simulink model "ARS1_2connection_k5"  (R2018a)
settings: Solver=VariableStepAuto  StartTime=0.0  StopTime=10.0  RelTol=1e-3
settings Model: Creator=moizh  LastModifiedBy=moizh

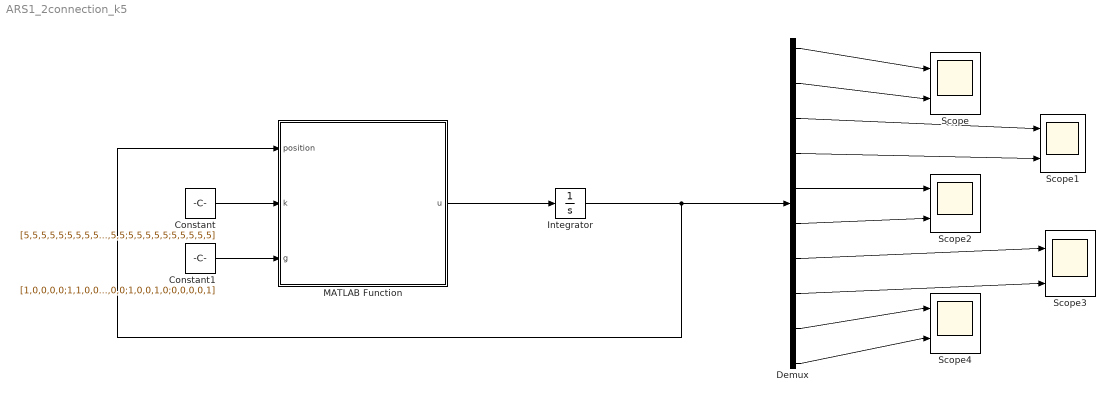
== system ARS1_2connection_k5 ==
  Constant : Constant  Value=[5,5,5,5,5;5,5,5,5,5;5,5,5,5,5;5,5,5,5,5;5,5,5,5,5]
  Constant1 : Constant  Value=[1,0,0,0,0;1,1,0,0,0;0,0,1,0,0;1,0,0,1,0;0,0,0,0,1]
  Demux : Demux  Outputs=10
  Integrator : Integrator  InitialCondition=[0;1.5;0;-1.5;-3;3;-3;0;-3;-3]
  MATLAB Function : MATLAB Function  TreatAsAtomicUnit=on
  Scope{,1..4} (5 alike) : Scope  NumInputPorts=2
  wires:
  Constant/1 -> MATLAB Function/2(k)
  Constant1/1 -> MATLAB Function/3(g)
  MATLAB Function/1(u) -> Integrator/1
  Integrator/1 -> MATLAB Function/1(position), Demux/1
  Demux/1 -> Scope/1
  Demux/2 -> Scope/2
  Demux/3 -> Scope1/1
  Demux/4 -> Scope1/2
  Demux/5 -> Scope2/1
  Demux/6 -> Scope2/2
  Demux/7 -> Scope3/1
  Demux/8 -> Scope3/2
  Demux/9 -> Scope4/1
  Demux/10 -> Scope4/2

== matlab function ARS1_2connection_k5/MATLAB Function ==
  data: position input; u output; k input; g input
function u = fcn(position,k,g)

 
a11 = -g(1,1)*k(1,1)-g(1,2)*k(1,2)-g(1,3)*k(1,3)-g(1,4)*k(1,4)-g(1,5)*k(1,5);
a12 = 0;
a13 = g(1,2)*k(1,2);
a14 = 0;
a15 = g(1,3)*k(1,3);
a16 = 0;
a17 = g(1,4)*k(1,4);
a18 = 0;
a19 = g(1,5)*k(1,5);
a110 = 0;

a21 = 0;
a22 = -g(1,1)*k(1,1)-g(1,2)*k(1,2)-g(1,3)*k(1,3)-g(1,4)*k(1,4)-g(1,5)*k(1,5);
a23 = 0;
a24 = g(1,2)*k(1,2);
a25 = 0;
a26 = g(1,3)*k(1,3);
a27 = 0;
a28 = g(1,4)*k(1,4);
a29 = 0;
a210 = g(1,5)*k(1,5);

a31 = g(2,1)*k(2,1);
a32 = 0;
a33 = -g(2,1)*k(2,1)-g(2,2)*k(2,2)-g(2,3)*k(2,3)-g(2,4)*k(2,4)-g(2,5)*k(2,5);
a34 = 0;
a35 = g(2,3)*k(2,3);
a36 = 0;
a37 = g(2,4)*k(2,4);
a38 = 0;
a39 = g(2,5)*k(2,5);
a310 = 0;

a41 = 0;
a42 = g(2,1)*k(2,1);
a43 = 0;
a44 = -g(2,1)*k(2,1)-g(2,2)*k(2,2)-g(2,3)*k(2,3)-g(2,4)*k(2,4)-g(2,5)*k(2,5);
a45 = 0;
a46 = g(2,3)*k(2,3);
a47 = 0;
a48 = g(2,4)*k(2,4);
a49 = 0;
a410 = g(2,5)*k(2,5);

a51 = g(3,1)*k(3,1);
a52 = 0;
a53 = g(3,2)*k(3,2);
a54 = 0;
a55 = -g(3,1)*k(3,1)-g(3,2)*k(3,2)-g(3,3)*k(3,3)-g(3,4)*k(3,4)-g(3,5)*k(3,5);
a56 = 0;
a57 = g(3,4)*k(3,4);
a58 = 0;
a59 = g(3,5)*k(3,5);
a510 = 0;

a61 = 0;
a62 = g(3,1)*k(3,1);
a63 = 0;
a64 = g(3,2)*k(3,2);
a65 = 0;
a66 = -g(3,1)*k(3,1)-g(3,2)*k(3,2)-g(3,3)*k(3,3)-g(3,4)*k(3,4)-g(3,5)*k(3,5);
a67 = 0;
a68 = g(3,4)*k(3,4);
a69 = 0;
a610 = g(3,5)*k(3,5);

a71 = g(4,1)*k(4,1);
a72 = 0;
a73 = g(4,2)*k(4,2);
a74 = 0;
a75 = g(4,3)*k(4,3);
a76 = 0;
a77 = -g(4,1)*k(4,1)-g(4,2)*k(4,2)-g(4,3)*k(4,3)-g(4,4)*k(4,4)-g(4,5)*k(4,5);
a78 = 0;
a79 = g(4,5)*k(4,5);
a710 = 0;

a81 = 0;
a82 = g(4,1)*k(4,1);
a83 = 0;
a84 = g(4,2)*k(4,2);
a85 = 0;
a86 = g(4,3)*k(4,3);
a87 = 0;
a88 = -g(4,1)*k(4,1)-g(4,2)*k(4,2)-g(4,3)*k(4,3)-g(4,4)*k(4,4)-g(4,5)*k(4,5);
a89 = 0;
a810 = g(4,5)*k(4,5);

a91 = g(5,1)*k(5,1);
a92 = 0;
a93 = g(5,2)*k(5,2);
a94 = 0;
a95 = g(5,3)*k(5,3);
a96 = 0;
a97 = g(5,4)*k(5,4);
a98 = 0;
a99 = -g(5,1)*k(5,1)-g(5,2)*k(5,2)-g(5,3)*k(5,3)-g(5,4)*k(5,4)-g(5,5)*k(5,5);
a910 = 0;

a101 = 0;
a102 = g(5,1)*k(5,1);
a103 = 0;
a104 = g(5,2)*k(5,2);
a105 = 0;
a106 = g(5,3)*k(5,3);
a107 = 0;
a108 = g(5,4)*k(5,4);
a109 = 0;
a1010 = -g(5,1)*k(5,1)-g(5,2)*k(5,2)-g(5,3)*k(5,3)-g(5,4)*k(5,4)-g(5,5)*k(5,5);
 
A = [a11 a12 a13 a14 a15 a16 a17 a18 a19 a110;
    a21 a22 a23 a24 a25 a26 a27 a28 a29 a210; 
    a31-g(2,1)*k(2,1) a32 a33+g(2,1)*k(2,1) a34 a35 a36 a37 a38 a39 a310; 
    a41 a42-g(2,1)*k(2,1) a43 a44+g(2,1)*k(2,1) a45 a46 a47 a48 a49 a410;
    a51 a52 a53 a54 a55 a56 a57 a58 a59 a510;
    a61 a62 a63 a64 a65 a66 a67 a68 a69 a610;
    a71-g(4,1)*k(4,1) a72 a73 a74 a75 a76 a77+g(4,1)*k(4,1) a78 a79 a710;
    a81 a82-g(4,1)*k(4,1) a83 a84 a85 a86 a87 a88+g(4,1)*k(4,1) a89 a810;
    a91 a92 a93 a94 a95 a96 a97 a98 a99 a910;
    a101 a102 a103 a104 a105 a106 a107 a108 a109 a1010];

B = [34;0;31;0;28;0;25;0;22;0]*5;

u = A * position + B;
